simulink model "FSFB_Const_Exp_2015"  (R2015a)
settings: Solver=ode1  StartTime=0.0  StopTime=90  FixedStep=0.001  RelTol=1e-3
values from neighbouring files (symbols this model uses):
  alpha1 = 10    [gains.m]
  alpha2 = 20    [gains.m]
  initialValues = [ 0 0 0 0 0]    [gains.m]
  Ke1 = 12    [gains.m]
  Ke2 = 24    [gains.m]
  Kr1 = 180    [gains.m]
  Kr2 = 50    [gains.m]
undefined symbols (not defined in the file or in its folder): Serial_Port, Standard_Devices
libraries: sldrtlib x2
settings Model: CovHtmlReporting=off  Creator=ezergeroglu  LastModifiedBy=Mesih
settings DataIOCC: SignalLoggingSaveFormat=ModelDataLogs  SignalLoggingName=sigsOut
settings OptimizationCC: BooleanDataType=off
settings DebuggingCC: SaveWithParameterizedLinksMsg=none  UnderspecifiedInitializationDetection=Classic  MergeDetectMultiDrivingBlocksExec=none  SignalResolutionControl=TryResolveAllWithWarning  MultiTaskDSMMsg=warning  MultiTaskCondExecSysMsg=none  SFUnexpectedBacktrackingDiag=error  SFNoUnconditionalDefaultTransitionDiag=error
settings HardwareCC: ProdBitPerPointer=64  ProdLargestAtomicFloat=Float  ProdIntDivRoundTo=Zero  ProdEndianess=LittleEndian  ProdHWDeviceType=Specified
settings RTWCC: Description=Simulink Desktop Real-Time  SystemTargetFile=rtwin.tlc  TemplateMakefile=rtwin.tmf  RTWCompilerOptimization=on
settings CodeAppCC: MaxIdLength=95
settings RTWinTargetCC: TargetPreCompLibLocation=C:\Program Files\MATLAB\R2020b\toolbox\sldrt\lib\win64  SupportVariableSizeSignals=on  UseToolchainInfoCompliant=off  ExtModeMexFile=sldrtext

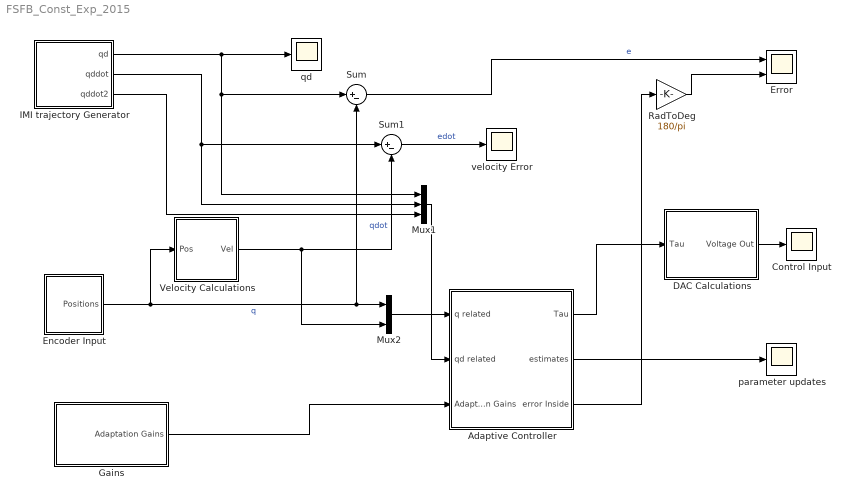
== system FSFB_Const_Exp_2015 ==
  Adaptive Controller : Subsystem
  Control Input : Scope
      settings: TimeRange=auto  ShowLegends=on  MaxDataPoints=5000  SaveName=InputsFromScope  YMin=-12.00000  YMax=12.00000  SampleTime=-1
  DAC Calculations : Subsystem
  Encoder Input : Subsystem
  Error : Scope  NumInputPorts=2
      settings: TimeRange=auto  MaxDataPoints=5000  SaveName=ErrorsFromScope  YMin=-0.06128~-3.12403  YMax=0.04841~2.39762  SampleTime=-1
  Gains : Subsystem
  IMI trajectory Generator : Subsystem  mask{ampl=[0.7  1.2], freq=[1.0 1.0]}
      mask prompts: ampl "Amplitute"; freq "Frequency"
  Mux1 : Mux  Inputs=3
  Mux2 : Mux  Inputs=2
  RadToDeg : Gain  Gain=180/pi  SaturateOnIntegerOverflow=on  OutDataTypeStr=Inherit: Same as input  ParamDataTypeStr=Inherit: Same as input
  Sum : Sum  Inputs=|+-  InputSameDT=on  SaturateOnIntegerOverflow=on  OutDataTypeStr=Inherit: Same as first input
  Sum1 : Sum  Inputs=|+-  InputSameDT=on  SaturateOnIntegerOverflow=on  OutDataTypeStr=Inherit: Same as first input
  Velocity Calculations : Subsystem
  parameter updates : Scope
      settings: TimeRange=auto  MaxDataPoints=5000  SaveName=ParamsFromScope  YMin=-15.5806  YMax=78.8377  SampleTime=-1
  qd : Scope
      settings: TimeRange=auto  MaxDataPoints=5000  SaveName=qdesFromScope  YMin=-1.5  YMax=1.5  SampleTime=-1
  velocity Error : Scope
      settings: TimeRange=auto  MaxDataPoints=5000  SaveToWorkspace=off  SaveName=ScopeData3  YMin=-0.4  YMax=0.35  SampleTime=-1
  wires:
  Sum/1 -> Error/1  "e"
  Encoder Input/1(Positions) -> Velocity Calculations/1(Pos), Sum/2, Mux2/1  "q"
  Velocity Calculations/1(Vel) -> Mux2/2, Sum1/2  "qdot"
  Sum1/1 -> velocity Error/1  "edot"
  Mux1/1 -> Adaptive Controller/2(qd related)
  Mux2/1 -> Adaptive Controller/1(q related)
  Adaptive Controller/2(estimates) -> parameter updates/1
  Adaptive Controller/3(error Inside) -> RadToDeg/1
  Gains/1(Adaptation Gains) -> Adaptive Controller/3(Adaptation Gains)
  IMI trajectory Generator/1(qd) -> Mux1/1, Sum/1, qd/1
  IMI trajectory Generator/2(qddot) -> Mux1/2, Sum1/1
  IMI trajectory Generator/3(qddot2) -> Mux1/3
  RadToDeg/1 -> Error/2
  Adaptive Controller/1(Tau) -> DAC Calculations/1(Tau)
  DAC Calculations/1(Voltage Out) -> Control Input/1

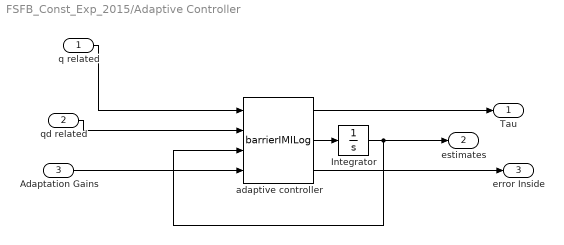
== system FSFB_Const_Exp_2015/Adaptive Controller ==
  q related : Inport
  qd related : Inport  Port=2
  Adaptation Gains : Inport  Port=3
  Integrator : Integrator  InitialCondition=initialValues
  adaptive controller : S-Function  FunctionName=barrierIMILog  Parameters=[Kr1, Kr2], [alpha1, alpha2], [Ke1, Ke2]  SFunctionDeploymentMode=off  EnableBusSupport=off
  Tau : Outport
  estimates : Outport  Port=2
  error Inside : Outport  Port=3
  wires:
  q related/1 -> adaptive controller/1
  qd related/1 -> adaptive controller/2
  adaptive controller/3 -> error Inside/1
  adaptive controller/2 -> Integrator/1
  Integrator/1 -> estimates/1, adaptive controller/3
  Adaptation Gains/1 -> adaptive controller/4
  adaptive controller/1 -> Tau/1

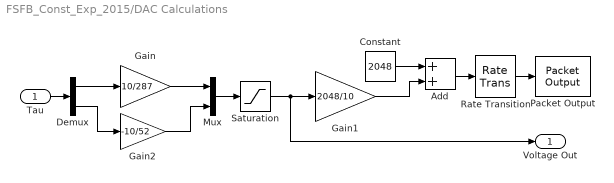
== system FSFB_Const_Exp_2015/DAC Calculations ==
  Tau : Inport
  Add : Sum  OutDataTypeStr=uint16
  Constant : Constant  Value=2048
  Demux : Demux  Outputs=2
  Gain : Gain  Gain=10/287
  Gain1 : Gain  Gain=2048/10
  Gain2 : Gain  Gain=-10/52
  Mux : Mux  Inputs=2
  Packet Output : sldrtlib/Packet Output  SampleTime=-1  MaxMissedTicks=1  ShowMissedTicks=off  YieldWhenWaiting=on  DrvName=Standard_Devices/Serial_Port  DrvAddress=2  DrvOptions=[256000 8 0 0 0 0 0 1]  PacketSize=4  DataTypes='2*uint16'  ShowReady=off  ShowError=off  PacketID=1  ByteOrder=1  InitialValue=[]  FinalValue=[]
      settings: AttributesFormatString=Serial Port [2]
  Rate Transition : RateTransition  Deterministic=off  OutPortSampleTimeOpt=Inherit  OutPortSampleTime=0.001
  Saturation : Saturate  UpperLimit=9.6  LowerLimit=-9.6
  Voltage Out : Outport
  wires:
  Add/1 -> Rate Transition/1
  Saturation/1 -> Voltage Out/1, Gain1/1
  Rate Transition/1 -> Packet Output/1
  Gain1/1 -> Add/2
  Constant/1 -> Add/1
  Mux/1 -> Saturation/1
  Tau/1 -> Demux/1
  Gain/1 -> Mux/1
  Demux/1 -> Gain/1
  Gain2/1 -> Mux/2
  Demux/2 -> Gain2/1

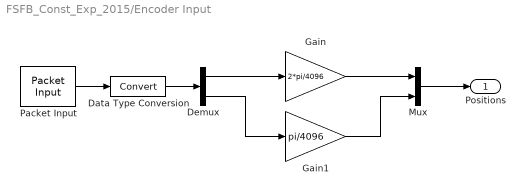
== system FSFB_Const_Exp_2015/Encoder Input ==
  Data Type Conversion : DataTypeConversion
  Demux : Demux  Outputs=2
  Gain : Gain  Gain=2*pi/4096
  Gain1 : Gain  Gain=pi/4096
  Mux : Mux  Inputs=2
  Packet Input : sldrtlib/Packet Input  SampleTime=-1  MaxMissedTicks=1  ShowMissedTicks=off  YieldWhenWaiting=on  DrvName=Standard_Devices/Serial_Port  DrvAddress=2  DrvOptions=[256000 8 0 0 0 0 0 0]  PacketSize=4  DataTypes='2*int16'  ShowReady=off  ShowError=off  PacketID=1  ByteOrder=1  ShowTimestamp=off
      settings: AttributesFormatString=Serial Port [2]
  Positions : Outport
  wires:
  Gain/1 -> Mux/1
  Mux/1 -> Positions/1
  Demux/1 -> Gain/1
  Data Type Conversion/1 -> Demux/1
  Packet Input/1 -> Data Type Conversion/1
  Demux/2 -> Gain1/1
  Gain1/1 -> Mux/2

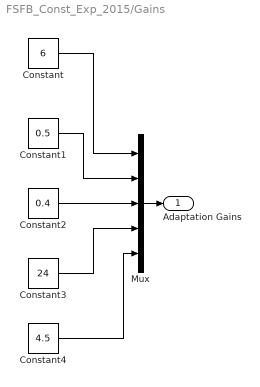
== system FSFB_Const_Exp_2015/Gains ==
  Constant : Constant  Value=6
  Constant1 : Constant  Value=0.5
  Constant2 : Constant  Value=0.4
  Constant3 : Constant  Value=24
  Constant4 : Constant  Value=4.5
  Mux : Mux  Inputs=5
  Adaptation Gains : Outport
  wires:
  Mux/1 -> Adaptation Gains/1
  Constant/1 -> Mux/1
  Constant1/1 -> Mux/2
  Constant2/1 -> Mux/3
  Constant3/1 -> Mux/4
  Constant4/1 -> Mux/5

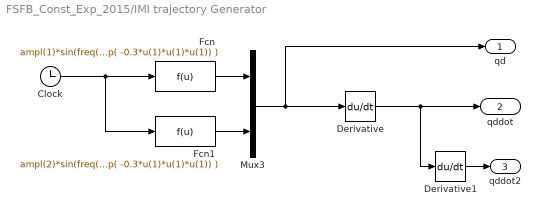
== system FSFB_Const_Exp_2015/IMI trajectory Generator ==
  Clock : Clock
  Derivative : Derivative
  Derivative1 : Derivative
  Fcn : Fcn  Expr=ampl(1)*sin(freq(1)*u(1))*( 1-exp( -0.3*u(1)*u(1)*u(1)) )
  Fcn1 : Fcn  Expr=ampl(2)*sin(freq(2)*u(1))*( 1-exp( -0.3*u(1)*u(1)*u(1)) )
  Mux3 : Mux  Inputs=2
  qd : Outport
  qddot : Outport  Port=2
  qddot2 : Outport  Port=3
  wires:
  Clock/1 -> Fcn/1, Fcn1/1
  Fcn/1 -> Mux3/1
  Fcn1/1 -> Mux3/2
  Mux3/1 -> Derivative/1, qd/1
  Derivative/1 -> Derivative1/1, qddot/1
  Derivative1/1 -> qddot2/1

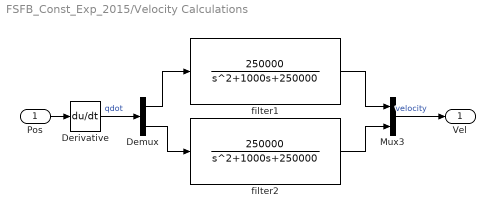
== system FSFB_Const_Exp_2015/Velocity Calculations ==
  Pos : Inport
  Demux : Demux  Outputs=2
  Derivative : Derivative
  Mux3 : Mux  Inputs=2
  filter1 : TransferFcn  Numerator=[250000]  Denominator=[1 1000 250000]
  filter2 : TransferFcn  Numerator=[250000]  Denominator=[1 1000 250000]
  Vel : Outport
  wires:
  Mux3/1 -> Vel/1  "velocity"
  Derivative/1 -> Demux/1  "qdot"
  filter1/1 -> Mux3/1
  Pos/1 -> Derivative/1
  filter2/1 -> Mux3/2
  Demux/1 -> filter1/1
  Demux/2 -> filter2/1
